simulink subsystem "ElectricalSystem1EMBevBattery"  (R2022b)
settings: Solver=VariableStepAuto  StartTime=0.0  StopTime=10.0  RelTol=1e-3
settings Model: ModifiedByFormat=The MathWorks, Inc.  Creator=The MathWorks, Inc.  LastModifiedBy=The MathWorks, Inc.
settings SolverCC: MaxZcPerStep=1
settings DebuggingCC: UnconnectedInputMsg=warning  UnconnectedOutputMsg=warning  UnconnectedLineMsg=warning
settings ModelReferenceCC: EnableRefExpFcnMdlSchedulingChecks=on
settings RTWCC: DLArmComputeVersion=19.05

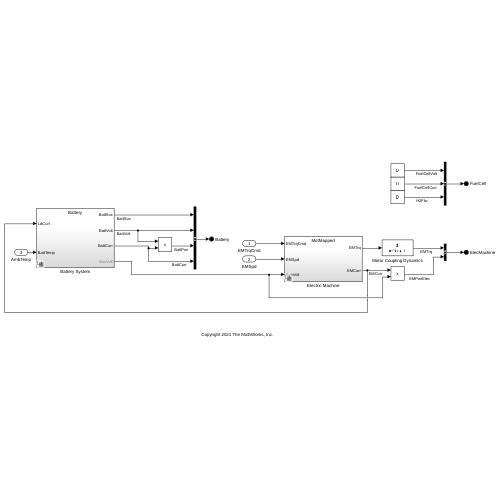
[thumbnail: Simulink's stored preview of the top-level diagram]
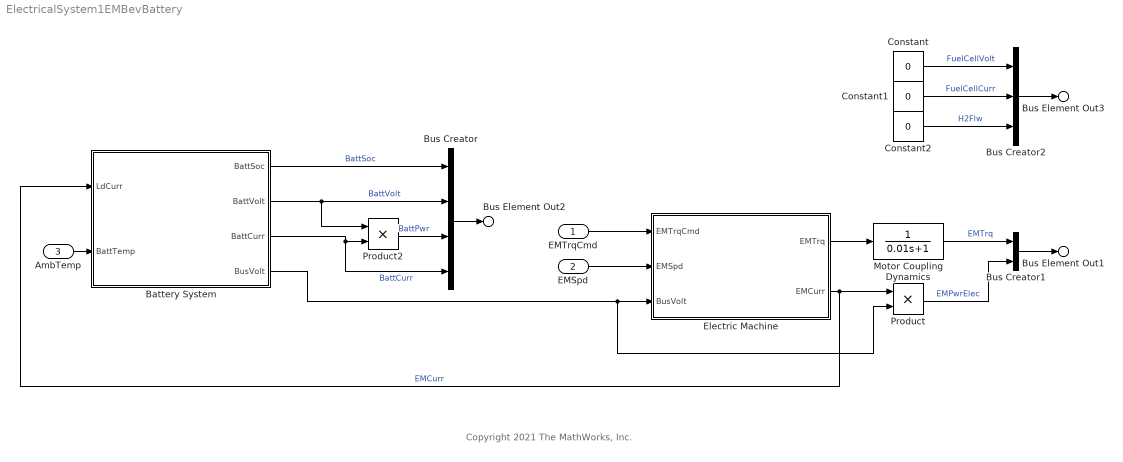
== system ElectricalSystem1EMBevBattery ==
  note: Copyright 2021 The MathWorks, Inc.
  EMTrqCmd : Inport
  EMSpd : Inport  Port=2
  AmbTemp : Inport  Port=3
  Battery System : Subsystem  Variant=on  VariantControlMode=label  LabelModeActiveChoice=0
  Bus Creator : BusCreator  Inputs=4
  Bus Creator1 : BusCreator  Inputs=2
  Bus Creator2 : BusCreator  Inputs=3
  Constant : Constant  Value=0  SampleTime=-1
  Constant1 : Constant  Value=0  SampleTime=-1
  Constant2 : Constant  Value=0  SampleTime=-1
  Electric Machine : Subsystem  Variant=on  VariantControlMode=label  LabelModeActiveChoice=0
  Motor Coupling Dynamics : TransferFcn  Denominator=[0.01 1]
  Product : Product
  Product2 : Product
  Bus Element Out2 : Outport  PortName=Battery
  Bus Element Out1 : Outport  Port=2  PortName=ElecMachine
  Bus Element Out3 : Outport  Port=3  PortName=FuelCell
  wires:
  Constant/1 -> Bus Creator2/1  "FuelCellVolt"
  Constant1/1 -> Bus Creator2/2  "FuelCellCurr"
  Constant2/1 -> Bus Creator2/3  "H2Flw"
  Bus Creator2/1 -> Bus Element Out3/1
  Bus Creator1/1 -> Bus Element Out1/1
  Product/1 -> Bus Creator1/2  "EMPwrElec"
  Bus Creator/1 -> Bus Element Out2/1
  Electric Machine/1(EMTrq) -> Motor Coupling Dynamics/1
  Motor Coupling Dynamics/1 -> Bus Creator1/1  "EMTrq"
  Battery System/4(BusVolt) -> Electric Machine/3(BusVolt), Product/2
  Battery System/3(BattCurr) -> Product2/2, Bus Creator/4  "BattCurr"
  Battery System/2(BattVolt) -> Product2/1, Bus Creator/2  "BattVolt"
  EMTrqCmd/1 -> Electric Machine/1(EMTrqCmd)
  Battery System/1(BattSoc) -> Bus Creator/1  "BattSoc"
  EMSpd/1 -> Electric Machine/2(EMSpd)
  Product2/1 -> Bus Creator/3  "BattPwr"
  Electric Machine/2(EMCurr) -> Battery System/1(LdCurr), Product/1  "EMCurr"
  AmbTemp/1 -> Battery System/2(BattTemp)

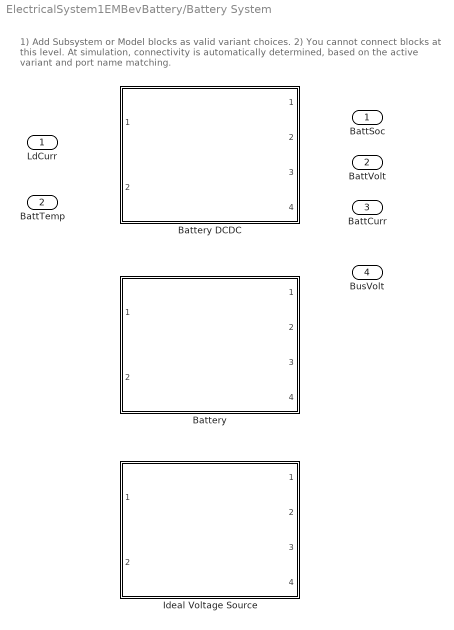
== system ElectricalSystem1EMBevBattery/Battery System ==
  note: 1) Add Subsystem or Model blocks as valid variant choices.
      | 2) You cannot connect blocks at this level. At simulation, connectivity is automatically
      | determined, based on the active variant and port name matching.
  LdCurr : Inport
  BattTemp : Inport  Port=2
  Battery : Subsystem  VariantControl=0  ReferencedSubsystem=Battery
  Battery DCDC : Subsystem  VariantControl=1  ReferencedSubsystem=BatteryDCDC
  Ideal Voltage Source : Subsystem  VariantControl=2  ReferencedSubsystem=IdealVoltageSource
  BattSoc : Outport  VectorParamsAs1DForOutWhenUnconnected=off
  BattVolt : Outport  Port=2  VectorParamsAs1DForOutWhenUnconnected=off
  BattCurr : Outport  Port=3  VectorParamsAs1DForOutWhenUnconnected=off
  BusVolt : Outport  Port=4  VectorParamsAs1DForOutWhenUnconnected=off

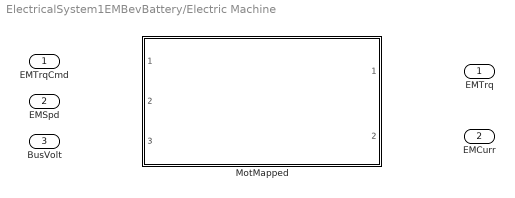
== system ElectricalSystem1EMBevBattery/Electric Machine ==
  EMTrqCmd : Inport
  EMSpd : Inport  Port=2
  BusVolt : Inport  Port=3
  MotMapped : Subsystem  VariantControl=0  ReferencedSubsystem=ElectricMachine1
  EMTrq : Outport  VectorParamsAs1DForOutWhenUnconnected=off
  EMCurr : Outport  Port=2  VectorParamsAs1DForOutWhenUnconnected=off
